simulink model "masa_resorte_nl"  (R2020b)
settings: Solver=VariableStepAuto  StartTime=0.0  StopTime=30  MaxStep=1e-3  RelTol=1e-3
settings Model: Creator=cmparedes  LastModifiedBy=Acer
settings SFSimCC: CustomCodeUndefinedFunction=UseInterfaceOnly

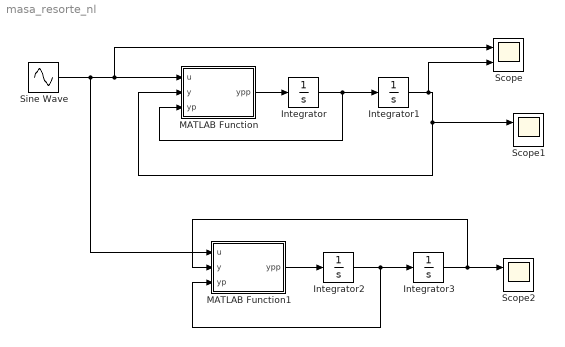
== system masa_resorte_nl ==
  Integrator{,1..3} (4 alike) : Integrator
  MATLAB Function : MATLAB Function  TreatAsAtomicUnit=on
  MATLAB Function1 : MATLAB Function  TreatAsAtomicUnit=on
  Scope : Scope  NumInputPorts=2
  Scope1 : Scope  NumInputPorts=2
  Scope2 : Scope  NumInputPorts=2
  Sine Wave : Sin  Frequency=10  SampleTime=0
  wires:
  MATLAB Function/1(ypp) -> Integrator/1
  Integrator/1 -> Integrator1/1, MATLAB Function/3(yp)
  Integrator1/1 -> Scope/2, Scope1/1, MATLAB Function/2(y)
  Sine Wave/1 -> MATLAB Function1/1(u), Scope/1, MATLAB Function/1(u)
  MATLAB Function1/1(ypp) -> Integrator2/1
  Integrator2/1 -> MATLAB Function1/3(yp), Integrator3/1
  Integrator3/1 -> Scope2/1, MATLAB Function1/2(y)

== matlab function masa_resorte_nl/MATLAB Function ==
  data: u input; ypp output; y input; yp input
function ypp = fcn(u,y,yp)
m=1;
c=1;
k=1;

a=10;

ypp = (u-c*yp+k*y+k*a^2*y^3)/m;

== matlab function masa_resorte_nl/MATLAB Function1 ==
  data: u input; ypp output; y input; yp input
function ypp = fcn(u,y,yp)
m=2;
c=1;
k=1;


ypp = (u-c*yp-k*y)/m;
